simulink library "CF3v2"  (R2013b)
settings: Solver=ode45  StartTime=0.0  StopTime=10.0  RelTol=1e-3
undefined symbols (not defined in the file): omega_n1_, zeta_
settings Model: Creator=Nam  LastModifiedBy=Nam

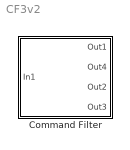
== system CF3v2 ==
  Command Filter : Subsystem  mask{Integrator1_init=0, omega_n=omega_n1_, zeta=zeta_}
      mask init:
      | zeta > 0
      | zeta <= 1
      mask DialogControl Control3_copy_copy Prompt: Initial value Integrator1
      mask DialogControl Control4 Prompt: omega_n
      mask DialogControl Control6 Prompt: zeta

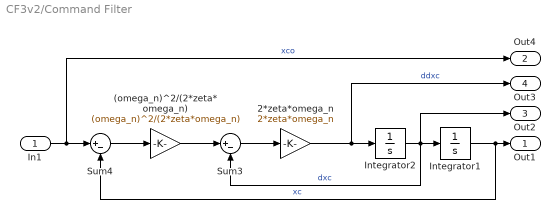
== system CF3v2/Command Filter ==
  In1 : Inport
  (omega_n)^2/(2*zeta*omega_n) : Gain  Gain=(omega_n)^2/(2*zeta*omega_n)
  2*zeta*omega_n : Gain  Gain=2*zeta*omega_n
  Integrator1 : Integrator  InitialCondition=Integrator1_init
  Integrator2 : Integrator
  Sum3 : Sum  Inputs=|+-
  Sum4 : Sum  Inputs=|+-
  Out1 : Outport
  Out4 : Outport  Port=2
  Out2 : Outport  Port=3
  Out3 : Outport  Port=4
  wires:
  2*zeta*omega_n/1 -> Integrator2/1, Out3/1  "ddxc"
  Integrator2/1 -> Sum3/2, Out2/1, Integrator1/1  "dxc"
  Integrator1/1 -> Sum4/2, Out1/1  "xc"
  Sum3/1 -> 2*zeta*omega_n/1
  Sum4/1 -> (omega_n)^2/(2*zeta*omega_n)/1
  (omega_n)^2/(2*zeta*omega_n)/1 -> Sum3/1
  In1/1 -> Out4/1, Sum4/1  "xco"
